simulink model "linear_longi"  (R2017b)
settings: Solver=VariableStepAuto  StartTime=0.0  StopTime=10.0  RelTol=1e-3
values from neighbouring files (symbols this model uses):
  A = A'    [c_l.m]    (also in c_m.m; c_n.m; c_x.m; c_z.m)
  altitude = input('Enter the altitude for the simulation (ft)  :  ')    [FindF16Dynamics.m]    (also in run_me.m = input(' altitude ( 0 ~ 40000 ft ) : '); trim_F16.m = alt)
  B = ssm_b( state_trim, state_dot_trim, control_trim, xcg )    [ssm_f16.m]    (also in thrust.m = B')
  C = ssm_c( state_trim, state_dot_trim, control_trim, xcg )    [ssm_f16.m]    (also in thrust.m = C')
  control_trim = u0    [find_trim.m]
  D = ssm_d( state_trim, state_dot_trim, control_trim, xcg )    [ssm_f16.m]
  state_trim = steady_state( state )    [find_trim.m]
  velocity = input('Enter the velocity for the simulation (ft/s):  ')    [FindF16Dynamics.m]    (also in run_me.m = input(' true velocity ( 350 ~ 1000 ft/sec ) : '); trim_F16.m = vel)
libraries: simulink x3
settings Model: Creator=monster  LastModifiedBy=monster

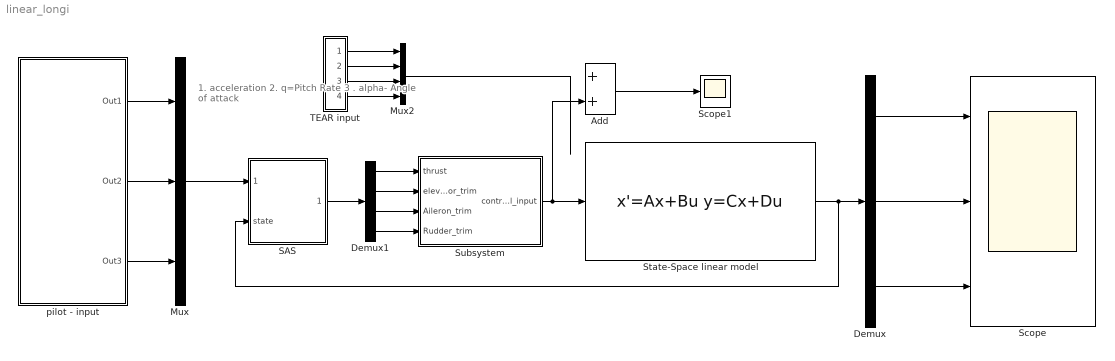
== system linear_longi ==
  note: 1. acceleration
      |
      | 2. q=Pitch Rate
      |
      | 3 . alpha- Angle of attack
  Add : Sum
  Demux : Demux  Outputs=3
  Demux1 : Demux
  Mux : Mux  Inputs=3
  Mux2 : Mux
  SAS : Subsystem
  Scope : Scope  NumInputPorts=3
  Scope1 : Scope
  "State-Space linear model " : StateSpace  A=A  B=B  C=C  D=D  InitialCondition=0
      mask Display: image('D:\Dropbox\M.eng\fall2017\flight control system\FDC\project\control surface.PNG');
  Subsystem : Subsystem
  TEAR input : Subsystem
  "pilot - input " : Subsystem
  wires:
  SAS/1(control_input) -> Demux1/1
  Demux1/2 -> Subsystem/2(elevator_trim)
  TEAR input/1(T) -> Mux2/1
  Mux2/1 -> ?
  Demux1/1 -> Subsystem/1(thrust)
  Demux1/3 -> Subsystem/3(Aileron_trim)
  Demux/3 -> Scope/3
  Subsystem/1(control_input) -> "State-Space linear model "/1, Add/2
  Demux1/4 -> Subsystem/4(Rudder_trim)
  Add/1 -> Scope1/1
  "pilot - input "/1(Out1) -> Mux/1
  TEAR input/3(A) -> Mux2/3
  Demux/1 -> Scope/1
  Demux/2 -> Scope/2
  TEAR input/4(R) -> Mux2/4
  TEAR input/2(E) -> Mux2/2
  Mux/1 -> SAS/1(reference)
  "State-Space linear model "/1 -> SAS/2(state), Demux/1
  "pilot - input "/2(Out2) -> Mux/2
  "pilot - input "/3(Out3) -> Mux/3

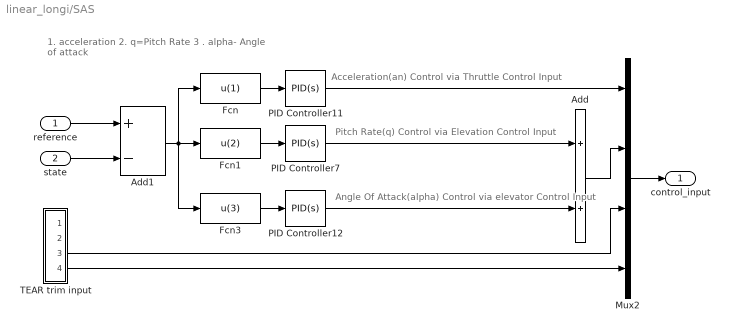
== system linear_longi/SAS ==
  note: Pitch Rate(q) Control via Elevation Control Input
  note: Acceleration(an) Control via Thruttle Control Input
  note: Angle Of Attack(alpha) Control via elevator Control Input
  note: 1. acceleration
      |
      | 2. q=Pitch Rate
      |
      | 3 . alpha- Angle of attack
  reference : Inport
  state : Inport  Port=2
  Add : Sum
  Add1 : Sum  Inputs=+-
  Fcn : Fcn  Expr=u(1)
  Fcn1 : Fcn  Expr=u(2)
  Fcn3 : Fcn  Expr=u(3)
  Mux2 : Mux
  PID Controller11 : simulink/Continuous/PID Controller  Controller=PID  TimeDomain=Continuous-time  SampleTime=-1  IntegratorMethod=Forward Euler  FilterMethod=Forward Euler  Form=Parallel  UseFilter=on  ControllerParametersSource=internal  P=13329483.1324469  I=392847306.175743  D=98980.5300334758  N=109037.560099343  InitialConditionSource=internal  InitialConditionForIntegrator=0  InitialConditionForFilter=0  ExternalReset=none  LimitOutput=off  UpperSaturationLimit=inf  LowerSaturationLimit=-inf  LinearizeAsGain=on  AntiWindupMode=none  Kb=1  TrackingMode=off  Kt=1  PParamMin=[]  PParamMax=[]  IParamMin=[]  IParamMax=[]  DParamMin=[]  DParamMax=[]  NParamMin=[]  NParamMax=[]  KbParamMin=[]  KbParamMax=[]  KtParamMin=[]  KtParamMax=[]  POutMin=[]  POutMax=[]  IOutMin=[]  IOutMax=[]  DOutMin=[]  DOutMax=[]  NOutMin=[]  NOutMax=[]  KbOutMin=[]  KbOutMax=[]  KtOutMin=[]  KtOutMax=[]  IntegratorOutMin=[]  IntegratorOutMax=[]  FilterOutMin=[]  FilterOutMax=[]  SumOutMin=[]  SumOutMax=[]  SumI1OutMin=[]  SumI1OutMax=[]  SumI2OutMin=[]  SumI2OutMax=[]  SumI3OutMin=[]  SumI3OutMax=[]  SumDOutMin=[]  SumDOutMax=[]  SaturationOutMin=[]  SaturationOutMax=[]  IntegratorContinuousStateAttributes=''  IntegratorStateMustResolveToSignalObject=off  IntegratorRTWStateStorageClass=Auto  FilterContinuousStateAttributes=''  FilterStateMustResolveToSignalObject=off  FilterRTWStateStorageClass=Auto  DifferentiatorICPrevScaledInput=0  DifferentiatorOutMin=[]  DifferentiatorOutMax=[]  InitialConditionSetting=State (most efficient)  FilterDiffOutCoefMin=[]  FilterDiffOutCoefMax=[]  SumDenOutMin=[]  SumDenOutMax=[]  SumNumOutMin=[]  SumNumOutMax=[]  ReciprocalOutMin=[]  ReciprocalOutMax=[]  DivideOutMin=[]  DivideOutMax=[]  TunerSelectOption=Transfer Function Based (PID Tuner App)
  PID Controller12 : simulink/Continuous/PID Controller  Controller=PID  TimeDomain=Continuous-time  SampleTime=-1  IntegratorMethod=Forward Euler  FilterMethod=Forward Euler  Form=Parallel  UseFilter=on  ControllerParametersSource=internal  P=-170.14183467408  I=-465.695324804371  D=-13.6839697818054  N=105.697856042613  InitialConditionSource=internal  InitialConditionForIntegrator=0  InitialConditionForFilter=0  ExternalReset=none  LimitOutput=off  UpperSaturationLimit=inf  LowerSaturationLimit=-inf  LinearizeAsGain=on  AntiWindupMode=none  Kb=1  TrackingMode=off  Kt=1  PParamMin=[]  PParamMax=[]  IParamMin=[]  IParamMax=[]  DParamMin=[]  DParamMax=[]  NParamMin=[]  NParamMax=[]  KbParamMin=[]  KbParamMax=[]  KtParamMin=[]  KtParamMax=[]  POutMin=[]  POutMax=[]  IOutMin=[]  IOutMax=[]  DOutMin=[]  DOutMax=[]  NOutMin=[]  NOutMax=[]  KbOutMin=[]  KbOutMax=[]  KtOutMin=[]  KtOutMax=[]  IntegratorOutMin=[]  IntegratorOutMax=[]  FilterOutMin=[]  FilterOutMax=[]  SumOutMin=[]  SumOutMax=[]  SumI1OutMin=[]  SumI1OutMax=[]  SumI2OutMin=[]  SumI2OutMax=[]  SumI3OutMin=[]  SumI3OutMax=[]  SumDOutMin=[]  SumDOutMax=[]  SaturationOutMin=[]  SaturationOutMax=[]  IntegratorContinuousStateAttributes=''  IntegratorStateMustResolveToSignalObject=off  IntegratorRTWStateStorageClass=Auto  FilterContinuousStateAttributes=''  FilterStateMustResolveToSignalObject=off  FilterRTWStateStorageClass=Auto  DifferentiatorICPrevScaledInput=0  DifferentiatorOutMin=[]  DifferentiatorOutMax=[]  InitialConditionSetting=State (most efficient)  FilterDiffOutCoefMin=[]  FilterDiffOutCoefMax=[]  SumDenOutMin=[]  SumDenOutMax=[]  SumNumOutMin=[]  SumNumOutMax=[]  ReciprocalOutMin=[]  ReciprocalOutMax=[]  DivideOutMin=[]  DivideOutMax=[]  TunerSelectOption=Transfer Function Based (PID Tuner App)
  PID Controller7 : simulink/Continuous/PID Controller  Controller=PID  TimeDomain=Continuous-time  SampleTime=-1  IntegratorMethod=Forward Euler  FilterMethod=Forward Euler  Form=Parallel  UseFilter=on  ControllerParametersSource=internal  P=-2409.99420452658  I=-41171.6281036838  D=-4.63151383685818  N=352.425457454863  InitialConditionSource=internal  InitialConditionForIntegrator=0  InitialConditionForFilter=0  ExternalReset=none  LimitOutput=off  UpperSaturationLimit=inf  LowerSaturationLimit=-inf  LinearizeAsGain=on  AntiWindupMode=none  Kb=1  TrackingMode=off  Kt=1  PParamMin=[]  PParamMax=[]  IParamMin=[]  IParamMax=[]  DParamMin=[]  DParamMax=[]  NParamMin=[]  NParamMax=[]  KbParamMin=[]  KbParamMax=[]  KtParamMin=[]  KtParamMax=[]  POutMin=[]  POutMax=[]  IOutMin=[]  IOutMax=[]  DOutMin=[]  DOutMax=[]  NOutMin=[]  NOutMax=[]  KbOutMin=[]  KbOutMax=[]  KtOutMin=[]  KtOutMax=[]  IntegratorOutMin=[]  IntegratorOutMax=[]  FilterOutMin=[]  FilterOutMax=[]  SumOutMin=[]  SumOutMax=[]  SumI1OutMin=[]  SumI1OutMax=[]  SumI2OutMin=[]  SumI2OutMax=[]  SumI3OutMin=[]  SumI3OutMax=[]  SumDOutMin=[]  SumDOutMax=[]  SaturationOutMin=[]  SaturationOutMax=[]  IntegratorContinuousStateAttributes=''  IntegratorStateMustResolveToSignalObject=off  IntegratorRTWStateStorageClass=Auto  FilterContinuousStateAttributes=''  FilterStateMustResolveToSignalObject=off  FilterRTWStateStorageClass=Auto  DifferentiatorICPrevScaledInput=0  DifferentiatorOutMin=[]  DifferentiatorOutMax=[]  InitialConditionSetting=State (most efficient)  FilterDiffOutCoefMin=[]  FilterDiffOutCoefMax=[]  SumDenOutMin=[]  SumDenOutMax=[]  SumNumOutMin=[]  SumNumOutMax=[]  ReciprocalOutMin=[]  ReciprocalOutMax=[]  DivideOutMin=[]  DivideOutMax=[]  TunerSelectOption=Transfer Function Based (PID Tuner App)
  TEAR trim input : Subsystem
  control_input : Outport
  wires:
  Mux2/1 -> control_input/1
  PID Controller11/1 -> Mux2/1
  Fcn3/1 -> PID Controller12/1
  PID Controller7/1 -> Add/1
  Fcn1/1 -> PID Controller7/1
  Fcn/1 -> PID Controller11/1
  Add/1 -> Mux2/2
  reference/1 -> Add1/1
  state/1 -> Add1/2
  Add1/1 -> Fcn3/1, Fcn1/1, Fcn/1
  PID Controller12/1 -> Add/2
  TEAR trim input/3(A) -> Mux2/3
  TEAR trim input/4(R) -> Mux2/4

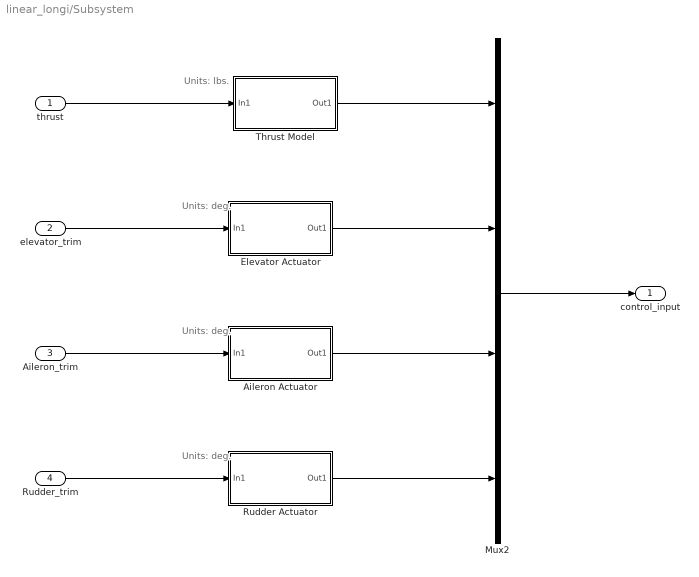
== system linear_longi/Subsystem ==
  note: Units: deg.
  note: Units: deg.
  note: Units: lbs.
  note: Units: deg.
  thrust : Inport
  elevator_trim : Inport  Port=2
  Aileron_trim : Inport  Port=3
  Rudder_trim : Inport  Port=4
  Aileron Actuator : Subsystem  AncestorBlock=F16_Actuator_Library/Aileron Actuator
  Elevator Actuator : Subsystem  AncestorBlock=F16_Actuator_Library/Elevator Actuator
  Mux2 : Mux
  Rudder Actuator : Subsystem  AncestorBlock=F16_Actuator_Library/Rudder Actuator
  Thrust Model : Subsystem  AncestorBlock=F16_Actuator_Library/Thrust Model
  control_input : Outport
  wires:
  thrust/1 -> Thrust Model/1(In1)
  Aileron Actuator/1(Out1) -> Mux2/3
  Rudder_trim/1 -> Rudder Actuator/1(In1)
  Elevator Actuator/1(Out1) -> Mux2/2
  Rudder Actuator/1(Out1) -> Mux2/4
  elevator_trim/1 -> Elevator Actuator/1(In1)
  Aileron_trim/1 -> Aileron Actuator/1(In1)
  Thrust Model/1(Out1) -> Mux2/1
  Mux2/1 -> control_input/1

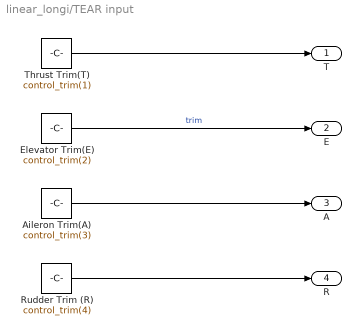
== system linear_longi/TEAR input ==
  "Aileron Trim(A) " : Constant  Value=control_trim(3)
  "Elevator Trim(E) " : Constant  Value=control_trim(2)  VectorParams1D=off
  Rudder Trim (R) : Constant  Value=control_trim(4)
  "Thrust Trim(T) " : Constant  Value=control_trim(1)
  T : Outport
  E : Outport  Port=2
  A : Outport  Port=3
  R : Outport  Port=4
  wires:
  "Aileron Trim(A) "/1 -> A/1
  "Elevator Trim(E) "/1 -> E/1  "trim"
  "Thrust Trim(T) "/1 -> T/1
  Rudder Trim (R)/1 -> R/1

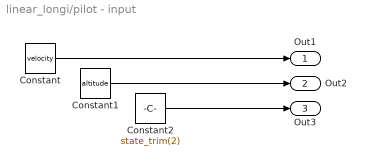
== system linear_longi/pilot - input  ==
  Constant : Constant  Value=velocity
  Constant1 : Constant  Value=altitude
  Constant2 : Constant  Value=state_trim(2)
  Out1 : Outport
  Out2 : Outport  Port=2
  Out3 : Outport  Port=3
  wires:
  Constant2/1 -> Out3/1
  Constant1/1 -> Out2/1
  Constant/1 -> Out1/1

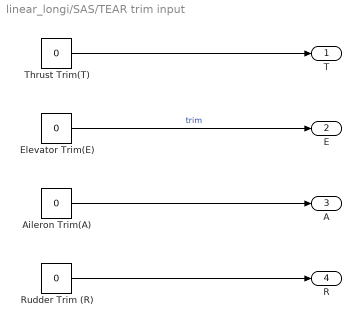
== system linear_longi/SAS/TEAR trim input ==
  "Aileron Trim(A) " : Constant  Value=0
  "Elevator Trim(E) " : Constant  Value=0  VectorParams1D=off
  Rudder Trim (R) : Constant  Value=0
  "Thrust Trim(T) " : Constant  Value=0
  T : Outport
  E : Outport  Port=2
  A : Outport  Port=3
  R : Outport  Port=4
  wires:
  "Aileron Trim(A) "/1 -> A/1
  "Elevator Trim(E) "/1 -> E/1  "trim"
  "Thrust Trim(T) "/1 -> T/1
  Rudder Trim (R)/1 -> R/1

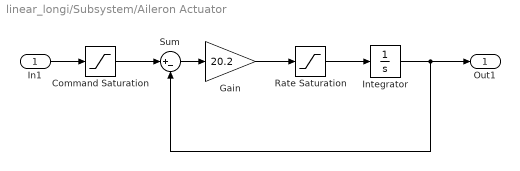
== system linear_longi/Subsystem/Aileron Actuator ==
  In1 : Inport
  Command Saturation : Saturate  UpperLimit=21.5  LowerLimit=-21.5
  Gain : Gain  Gain=20.2  SaturateOnIntegerOverflow=on  OutDataTypeStr=Inherit: Same as input  ParamDataTypeStr=Inherit: Same as input
  "Integrator " : Integrator  UpperSaturationLimit=21.5  LowerSaturationLimit=-21.5
  Rate Saturation : Saturate  UpperLimit=80  LowerLimit=-80
  Sum : Sum  Inputs=|+-  SaturateOnIntegerOverflow=on  InputSameDT=on  OutDataTypeStr=Inherit: Same as first input
  Out1 : Outport
  wires:
  "Integrator "/1 -> Sum/2, Out1/1
  Rate Saturation/1 -> "Integrator "/1
  Gain/1 -> Rate Saturation/1
  Sum/1 -> Gain/1
  Command Saturation/1 -> Sum/1
  In1/1 -> Command Saturation/1

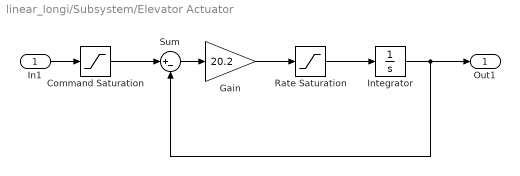
== system linear_longi/Subsystem/Elevator Actuator ==
  In1 : Inport
  Command Saturation : Saturate  UpperLimit=25  LowerLimit=-25
  Gain : Gain  Gain=20.2  SaturateOnIntegerOverflow=on  OutDataTypeStr=Inherit: Same as input  ParamDataTypeStr=Inherit: Same as input
  "Integrator " : Integrator  UpperSaturationLimit=25  LowerSaturationLimit=-25
  Rate Saturation : Saturate  UpperLimit=60  LowerLimit=-60
  Sum : Sum  Inputs=|+-  SaturateOnIntegerOverflow=on  InputSameDT=on  OutDataTypeStr=Inherit: Same as first input
  Out1 : Outport
  wires:
  "Integrator "/1 -> Sum/2, Out1/1
  Rate Saturation/1 -> "Integrator "/1
  Gain/1 -> Rate Saturation/1
  Sum/1 -> Gain/1
  Command Saturation/1 -> Sum/1
  In1/1 -> Command Saturation/1

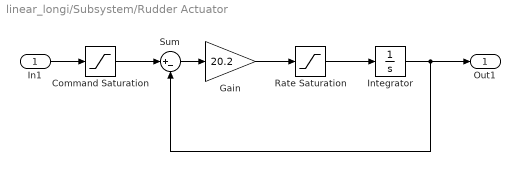
== system linear_longi/Subsystem/Rudder Actuator ==
  In1 : Inport
  Command Saturation : Saturate  UpperLimit=30  LowerLimit=-30
  Gain : Gain  Gain=20.2  SaturateOnIntegerOverflow=on  OutDataTypeStr=Inherit: Same as input  ParamDataTypeStr=Inherit: Same as input
  "Integrator " : Integrator  UpperSaturationLimit=30  LowerSaturationLimit=-30
  Rate Saturation : Saturate  UpperLimit=120  LowerLimit=-120
  Sum : Sum  Inputs=|+-  SaturateOnIntegerOverflow=on  InputSameDT=on  OutDataTypeStr=Inherit: Same as first input
  Out1 : Outport
  wires:
  "Integrator "/1 -> Sum/2, Out1/1
  Rate Saturation/1 -> "Integrator "/1
  Gain/1 -> Rate Saturation/1
  Sum/1 -> Gain/1
  Command Saturation/1 -> Sum/1
  In1/1 -> Command Saturation/1

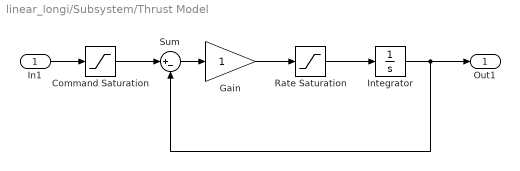
== system linear_longi/Subsystem/Thrust Model ==
  In1 : Inport
  Command Saturation : Saturate  UpperLimit=19000  LowerLimit=1000
  Gain : Gain  SaturateOnIntegerOverflow=on  OutDataTypeStr=Inherit: Same as input  ParamDataTypeStr=Inherit: Same as input
  "Integrator " : Integrator  UpperSaturationLimit=30  LowerSaturationLimit=-30
  Rate Saturation : Saturate  UpperLimit=10000  LowerLimit=-10000
  Sum : Sum  Inputs=|+-  SaturateOnIntegerOverflow=on  InputSameDT=on  OutDataTypeStr=Inherit: Same as first input
  Out1 : Outport
  wires:
  "Integrator "/1 -> Sum/2, Out1/1
  Rate Saturation/1 -> "Integrator "/1
  Gain/1 -> Rate Saturation/1
  Sum/1 -> Gain/1
  Command Saturation/1 -> Sum/1
  In1/1 -> Command Saturation/1
